simulink model "meu_esboco"  (R2017a)
settings: Solver=VariableStepAuto  StartTime=0.0  StopTime=30  RelTol=1e-3
values from neighbouring files (symbols this model uses):
  K = acker(A,B,J)    [principal.m]
libraries: simulink x8
settings Model: Creator=dscat  LastModifiedBy=dscat

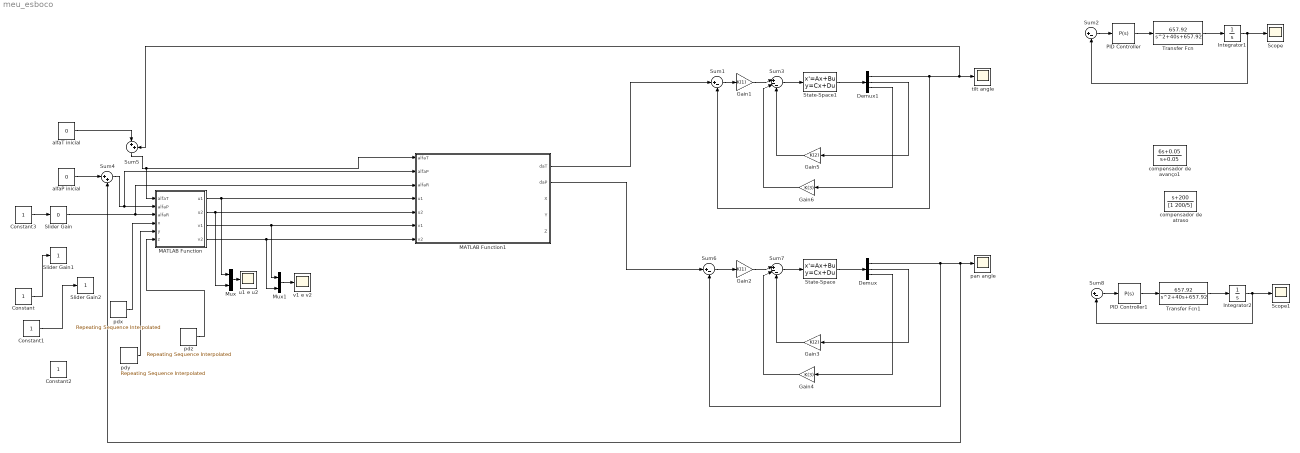
== system meu_esboco ==
  Constant{,1..3} (4 alike) : Constant
  Demux : Demux  Outputs=3
  Demux1 : Demux  Outputs=3
  Gain1 : Gain  Gain=K(1)
  Gain2 : Gain  Gain=K(1)
  Gain3 : Gain  Gain=K(2)
  Gain4 : Gain  Gain=K(3)
  Gain5 : Gain  Gain=K(2)
  Gain6 : Gain  Gain=K(3)
  Integrator1 : Integrator
  Integrator2 : Integrator
  MATLAB Function : MATLAB Function  TreatAsAtomicUnit=on
  MATLAB Function1 : MATLAB Function  TreatAsAtomicUnit=on
  Mux : Mux  Inputs=2
  Mux1 : Mux  Inputs=2
  PID Controller : simulink/Continuous/PID Controller  Controller=P  TimeDomain=Continuous-time  SampleTime=-1  IntegratorMethod=Forward Euler  FilterMethod=Forward Euler  Form=Parallel  UseFilter=on  ControllerParametersSource=internal  P=6.5  I=4.329  D=1.846  N=3518  InitialConditionSource=internal  InitialConditionForIntegrator=0  InitialConditionForFilter=0  ExternalReset=none  LimitOutput=off  UpperSaturationLimit=inf  LowerSaturationLimit=-inf  LinearizeAsGain=on  AntiWindupMode=none  Kb=1  TrackingMode=off  Kt=1  PParamMin=[]  PParamMax=[]  IParamMin=[]  IParamMax=[]  DParamMin=[]  DParamMax=[]  NParamMin=[]  NParamMax=[]  KbParamMin=[]  KbParamMax=[]  KtParamMin=[]  KtParamMax=[]  POutMin=[]  POutMax=[]  IOutMin=[]  IOutMax=[]  DOutMin=[]  DOutMax=[]  NOutMin=[]  NOutMax=[]  KbOutMin=[]  KbOutMax=[]  KtOutMin=[]  KtOutMax=[]  IntegratorOutMin=[]  IntegratorOutMax=[]  FilterOutMin=[]  FilterOutMax=[]  SumOutMin=[]  SumOutMax=[]  SumI1OutMin=[]  SumI1OutMax=[]  SumI2OutMin=[]  SumI2OutMax=[]  SumI3OutMin=[]  SumI3OutMax=[]  SumDOutMin=[]  SumDOutMax=[]  SaturationOutMin=[]  SaturationOutMax=[]  IntegratorContinuousStateAttributes=''  IntegratorStateMustResolveToSignalObject=off  IntegratorRTWStateStorageClass=Auto  FilterContinuousStateAttributes=''  FilterStateMustResolveToSignalObject=off  FilterRTWStateStorageClass=Auto  DifferentiatorICPrevScaledInput=0  DifferentiatorOutMin=[]  DifferentiatorOutMax=[]  InitialConditionSetting=State (most efficient)
  PID Controller1 : simulink/Continuous/PID Controller  Controller=P  TimeDomain=Continuous-time  SampleTime=-1  IntegratorMethod=Forward Euler  FilterMethod=Forward Euler  Form=Parallel  UseFilter=on  ControllerParametersSource=internal  P=6.5  I=4.329  D=1.846  N=3518  InitialConditionSource=internal  InitialConditionForIntegrator=0  InitialConditionForFilter=0  ExternalReset=none  LimitOutput=off  UpperSaturationLimit=inf  LowerSaturationLimit=-inf  LinearizeAsGain=on  AntiWindupMode=none  Kb=1  TrackingMode=off  Kt=1  PParamMin=[]  PParamMax=[]  IParamMin=[]  IParamMax=[]  DParamMin=[]  DParamMax=[]  NParamMin=[]  NParamMax=[]  KbParamMin=[]  KbParamMax=[]  KtParamMin=[]  KtParamMax=[]  POutMin=[]  POutMax=[]  IOutMin=[]  IOutMax=[]  DOutMin=[]  DOutMax=[]  NOutMin=[]  NOutMax=[]  KbOutMin=[]  KbOutMax=[]  KtOutMin=[]  KtOutMax=[]  IntegratorOutMin=[]  IntegratorOutMax=[]  FilterOutMin=[]  FilterOutMax=[]  SumOutMin=[]  SumOutMax=[]  SumI1OutMin=[]  SumI1OutMax=[]  SumI2OutMin=[]  SumI2OutMax=[]  SumI3OutMin=[]  SumI3OutMax=[]  SumDOutMin=[]  SumDOutMax=[]  SaturationOutMin=[]  SaturationOutMax=[]  IntegratorContinuousStateAttributes=''  IntegratorStateMustResolveToSignalObject=off  IntegratorRTWStateStorageClass=Auto  FilterContinuousStateAttributes=''  FilterStateMustResolveToSignalObject=off  FilterRTWStateStorageClass=Auto  DifferentiatorICPrevScaledInput=0  DifferentiatorOutMin=[]  DifferentiatorOutMax=[]  InitialConditionSetting=State (most efficient)
  Scope : Scope
  Scope1 : Scope
  Slider Gain : simulink/Math Operations/Slider Gain  gain=0  low=-3.14  high=3.14
  Slider Gain1 : simulink/Math Operations/Slider Gain  gain=1  low=-5  high=5
  Slider Gain2 : simulink/Math Operations/Slider Gain  gain=1  low=-5  high=5
  State-Space : StateSpace  A=[0 657.92 0; 0 0 1; 0 -657.92 -40]  B=[0; 0; 1]  C=[1 0 0; 0 1 0; 0 0 1]  D=[0; 0; 0]  X0=0
  State-Space1 : StateSpace  A=[0 657.92 0; 0 0 1; 0 -657.92 -40]  B=[0; 0; 1]  C=[1 0 0; 0 1 0; 0 0 1]  D=[0; 0; 0]  X0=0
  Sum{1..2,6,8} (4 alike) : Sum  Inputs=|+-
  Sum3 : Sum  Inputs=|+--
  Sum4 : Sum  Inputs=|++
  Sum5 : Sum  Inputs=|++
  Sum7 : Sum  Inputs=|+--
  Transfer Fcn : TransferFcn  Numerator=[657.92]  Denominator=[1 40 657.92]
  Transfer Fcn1 : TransferFcn  Numerator=[657.92]  Denominator=[1 40 657.92]
  alfaP inicial : Constant  Value=0
  alfaT inicial : Constant  Value=0
  compensador de atraso : TransferFcn  Numerator=[1 200]  Denominator=[1 200/5]
  compensador de avanço1 : TransferFcn  Numerator=[6 0.05]  Denominator=[1 0.05]
  pan angle : Scope
  pdx : simulink/Sources/Repeating Sequence Interpolated  OutValues=pdx  TimeValues=t  LookUpMeth=Interpolation-Use End Values  tsamp=0.01  OutMin=[]  OutMax=[]  OutDataTypeStr=double  OutputDataTypeScalingMode=double  OutDataType=fixdt(0,8)  OutScaling=2^-10
  pdy : simulink/Sources/Repeating Sequence Interpolated  OutValues=pdy  TimeValues=t  LookUpMeth=Interpolation-Use End Values  tsamp=0.01  OutMin=[]  OutMax=[]  OutDataTypeStr=double  OutputDataTypeScalingMode=double  OutDataType=fixdt(0,8)  OutScaling=2^-10
  pdz : simulink/Sources/Repeating Sequence Interpolated  OutValues=pdz  TimeValues=t  LookUpMeth=Interpolation-Use End Values  tsamp=0.01  OutMin=[]  OutMax=[]  OutDataTypeStr=double  OutputDataTypeScalingMode=double  OutDataType=fixdt(0,8)  OutScaling=2^-10
  tilt angle : Scope
  u1 e u2 : Scope
  v1 e v2 : Scope
  wires:
  MATLAB Function/1(u1) -> MATLAB Function1/4(u1), Mux/1
  MATLAB Function/2(u2) -> MATLAB Function1/5(u2), Mux/2
  Sum5/1 -> MATLAB Function1/1(alfaT), MATLAB Function/1(alfaT)
  Sum4/1 -> MATLAB Function1/2(alfaP), MATLAB Function/2(alfaP)
  Slider Gain/1 -> MATLAB Function1/3(alfaR), MATLAB Function/3(alfaR)
  Constant/1 -> Slider Gain1/1
  Constant1/1 -> Slider Gain2/1
  alfaP inicial/1 -> Sum4/1
  alfaT inicial/1 -> Sum5/1
  Mux/1 -> u1 e u2/1
  Mux1/1 -> v1 e v2/1
  MATLAB Function/3(v1) -> Mux1/1, MATLAB Function1/6(v1)
  MATLAB Function/4(v2) -> Mux1/2, MATLAB Function1/7(v2)
  Demux/3 -> Gain4/1
  State-Space/1 -> Demux/1
  Demux/2 -> Gain3/1
  Gain4/1 -> Sum7/2
  Sum7/1 -> State-Space/1
  Demux/1 -> Sum6/2, Sum4/2, pan angle/1
  Gain3/1 -> Sum7/3
  Gain2/1 -> Sum7/1
  Gain1/1 -> Sum3/1
  Sum3/1 -> State-Space1/1
  Gain6/1 -> Sum3/2
  State-Space1/1 -> Demux1/1
  Gain5/1 -> Sum3/3
  Demux1/2 -> Gain5/1
  Demux1/3 -> Gain6/1
  Demux1/1 -> Sum1/2, Sum5/2, tilt angle/1
  Constant3/1 -> Slider Gain/1
  Sum1/1 -> Gain1/1
  Sum6/1 -> Gain2/1
  pdx/1 -> MATLAB Function/4(x)
  pdy/1 -> MATLAB Function/5(y)
  pdz/1 -> MATLAB Function/6(z)
  Transfer Fcn/1 -> Integrator1/1
  Integrator1/1 -> Sum2/2, Scope/1
  PID Controller/1 -> Transfer Fcn/1
  Sum2/1 -> PID Controller/1
  PID Controller1/1 -> Transfer Fcn1/1
  Sum8/1 -> PID Controller1/1
  Transfer Fcn1/1 -> Integrator2/1
  Integrator2/1 -> Sum8/2, Scope1/1
  MATLAB Function1/1(daT) -> Sum1/1
  MATLAB Function1/2(daP) -> Sum6/1

== matlab function meu_esboco/MATLAB Function1 ==
  data: alfaT input; daT output; alfaP input; alfaR input; u1 input; u2 input; v1 input; v2 input; daP output; X output; Y output; Z output
function [daT, daP, X,Y,Z  ] = image2real( alfaT,alfaP,alfaR, u1,u2,v1,v2)
% daT -> Delta Alfa Tilt
% daP -> Delta Alfa Pan
% AlfaR -> Lido dos encoders


l = 0.15; %Tamanho do alvo (m) 
f = 664;

X = (l*(f*cos(alfaP-alfaR) - u2*sin(alfaP-alfaR))*(- cos(alfaP-alfaR)*sin(alfaP-alfaR)*f^2 + (u1 - cos(alfaP-alfaR)^2*(u1 + u2))*f + u1*u2*cos(alfaP-alfaR)*sin(alfaP-alfaR)))/(f*(u2*cos(alfaP-alfaR) + f*sin(alfaP-alfaR))*(u1 - u2));

%  X = (l*(f*cos(alfaT) - v2*sin(alfaT))*(- cos(alfaT)*sin(alfaT)*f^2 + (v1 - cos(alfaT)^2*(v1 + v2))*f + v1*v2*cos(alfaT)*sin(alfaT)))/(f*(f*sin(alfaT) + v2*cos(alfaT))*(v1 - v2));

Y = -(l*(2*cos(alfaP-alfaR)*sin(alfaP-alfaR)*f^2 + (u1 + u2)*(2*cos(alfaP-alfaR)^2 - 1)*f - 2*u1*u2*cos(alfaP-alfaR)*sin(alfaP-alfaR)))/(2*f*(u1 - u2));

Z  = -(l*(2*cos(alfaT)*sin(alfaT)*f^2 + (v1 + v2)*(2*cos(alfaT)^2 - 1)*f - 2*v1*v2*cos(alfaT)*sin(alfaT)))/(2*f*(v1 - v2));
 
daP = double(atan(Y/X)-alfaR);
daT = double(atan(Z/(sqrt((X)^2+(Y)^2))));


end

== matlab function meu_esboco/MATLAB Function ==
  data: alfaT input; u1 output; alfaP input; alfaR input; x input; y input; z input; u2 output; v1 output; v2 output
function [u1, u2, v1, v2] = real2image(alfaT,alfaP,alfaR,x,y,z)
L = 0.15;
f = 664;
u1 = f*(-sin(alfaP-alfaR)*(-x)+cos(alfaP-alfaR)*((L/2)-y))/((cos(alfaP-alfaR)*(-x)+sin(alfaP-alfaR)*((L/2)-y)));
u2 = f*(-sin(alfaP-alfaR)*(-x)+cos(alfaP-alfaR)*((-L/2)-y))/((cos(alfaP-alfaR)*(-x)+sin(alfaP-alfaR)*((-L/2)-y)));
v1 = f*(-sin(alfaT)*(-x)+cos(alfaT)*((L/2)-z))/((cos(alfaT)*(-x)+sin(alfaT)*((L/2)-z)));
v2 = f*(-sin(alfaT)*(-x)+cos(alfaT)*((-L/2)-z))/((cos(alfaT)*(-x)+sin(alfaT)*((-L/2)-z)));

end
